simulink model "Lab5"  (R2015a)
settings: Solver=ode8  StartTime=0.0  StopTime=300  FixedStep=0.001  RelTol=1e-3
values from neighbouring files (symbols this model uses):
  B = [2,5,3,6]    [Lab1.m]    (also in cruise_speed.m = 30; mass_spring.m = 30)
  K = 15    [mass_spring.m]
  M = 750    [cruise_speed.m]    (also in mass_spring.m = 705)
undefined symbols (not defined in the file or in its folder): F
settings Model: Creator=Bilal  LastModifiedBy=Bilal

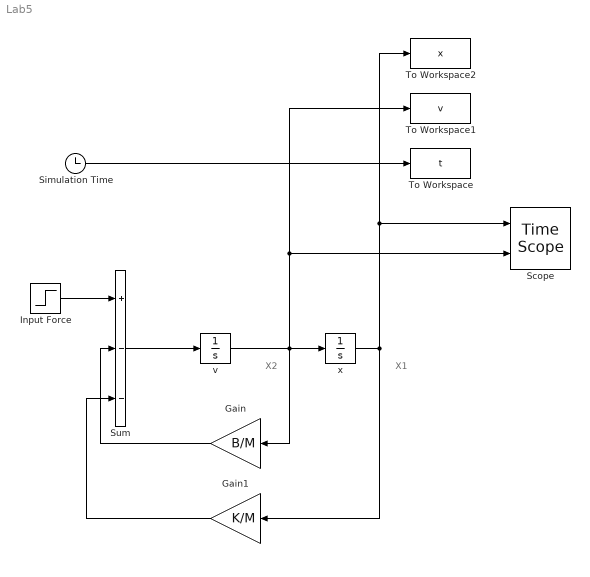
== system Lab5 ==
  note: X1
  note: X2
  Gain : Gain  Gain=B/M
  Gain1 : Gain  Gain=K/M
  Input Force : Step  Time=0  After=F/M  SampleTime=0
  Scope : TimeScope  NumInputPorts=2
  Simulation Time : Clock
  Sum : Sum  Inputs=+--
  To Workspace : ToWorkspace  VariableName=t  SampleTime=-1
      settings: Save2DSignal=2-D array (concatenate along first dimension)
  To Workspace1 : ToWorkspace  VariableName=v  SampleTime=-1
      settings: Save2DSignal=2-D array (concatenate along first dimension)
  To Workspace2 : ToWorkspace  VariableName=x  SampleTime=-1
      settings: Save2DSignal=2-D array (concatenate along first dimension)
  v : Integrator
  x : Integrator
  wires:
  v/1 -> To Workspace1/1, Scope/2, Gain/1, x/1
  Sum/1 -> v/1
  Input Force/1 -> Sum/1
  x/1 -> Gain1/1, To Workspace2/1, Scope/1
  Gain/1 -> Sum/2
  Gain1/1 -> Sum/3
  Simulation Time/1 -> To Workspace/1
